simulink model "CDM"  (R2022b)
settings: Solver=FixedStepAuto  StartTime=0.0  StopTime=55.0  FixedStep=0.001  RelTol=1e-3
values from neighbouring files (symbols this model uses):
  a = K - (2 * M) / (dt)^2    [CDM_ACC_or_Disp_Input.m]    (also in Final_10DOFs_RTHS.m; ThreeDOFs_CDM_Dampling.m; ThreeDOFs_CDM_substructure.m; ThreeDOFs_Dampling.m)
  ACC_el = ACC_el(1:10000,:)    [ThreeDOFs_Dampling.m]    (also in ThreeDOFs_noDampling.m; multiDOFs_CDM_highspeed_Dampling.m = ACC_el(1:2000,:); multiDOFs_auto_for_loop.m = ACC_el(1:1000,:); multiDOFs_highspeed.m = ACC_el(1:1000,:))
  b = M/dt^2 - C/(2*dt)    [CDM_ACC_or_Disp_Input.m]    (also in Final_10DOFs_RTHS.m; ThreeDOFs_CDM_Dampling.m; ThreeDOFs_CDM_substructure.m; ThreeDOFs_Dampling.m)
  diagM = diag(M)    [CDM_ACC_or_Disp_Input.m]    (also in Final_10DOFs_RTHS.m; ThreeDOFs_CDM_Dampling.m; ThreeDOFs_CDM_substructure.m; ThreeDOFs_Dampling.m)
  Ke_inv = inv(Ke)    [structure_2DOFs.m]
libraries: dspsrcs4 x1
settings Model: Creator=dongxh  LastModifiedBy=dongxh

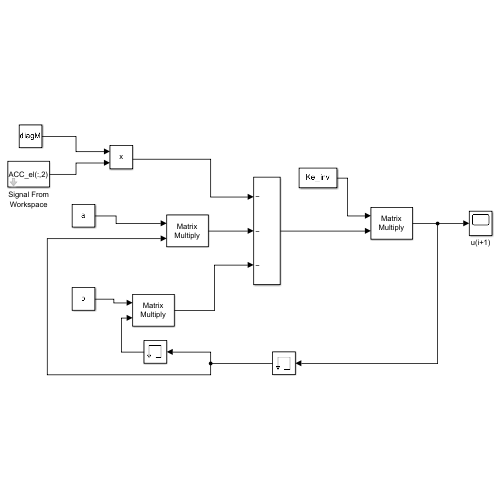
[thumbnail: Simulink's stored preview of the top-level diagram]
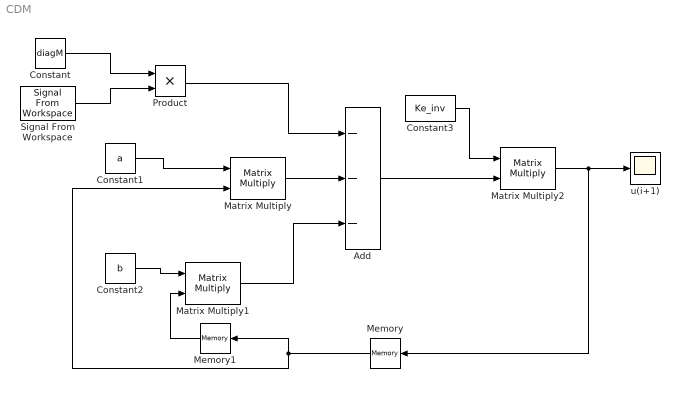
== system CDM ==
  Add : Sum  Inputs=---
  Constant : Constant  Value=diagM  VectorParams1D=off
  Constant1 : Constant  Value=a  VectorParams1D=off
  Constant2 : Constant  Value=b  VectorParams1D=off
  Constant3 : Constant  Value=Ke_inv  VectorParams1D=off
  Matrix Multiply : Product  Multiplication=Matrix(*)
  Matrix Multiply1 : Product  Multiplication=Matrix(*)
  Matrix Multiply2 : Product  Multiplication=Matrix(*)
  Memory : Memory
  Memory1 : Memory
  Product : Product
  Signal From Workspace : dspsrcs4/Signal From Workspace  X=ACC_el(:,2)  Ts=0.001  nsamps=1  OutputAfterFinalValue=Setting to zero  ignoreOrWarnInputAndFrameLengths=off  OutputFrames=off
  u(i+1) : Scope
  wires:
  Constant/1 -> Product/1
  Signal From Workspace/1 -> Product/2
  Constant1/1 -> Matrix Multiply/1
  Product/1 -> Add/1
  Add/1 -> Matrix Multiply2/2
  Matrix Multiply2/1 -> u(i+1)/1, Memory/1
  Memory/1 -> Matrix Multiply/2, Memory1/1
  Matrix Multiply/1 -> Add/2
  Constant2/1 -> Matrix Multiply1/1
  Matrix Multiply1/1 -> Add/3
  Constant3/1 -> Matrix Multiply2/1
  Memory1/1 -> Matrix Multiply1/2
